simulink model "simulink_qbat_model"  (R2020b)
settings: Solver=ode4  StartTime=0.0  StopTime=1800  FixedStep=0.01  MaxStep=10  MinStep=0.1  RelTol=1e-3
model workspace (MAT data in the model file):
  air_initial_temperature = 25
  coolant_initial_temperature = 25
  electro_model = struct()
  fem_model = struct()
  heat_dt = 1
  initial_SOC = 0.8
  max_res = 0.001
  n_fv_gradient_subiters = 20
  n_subiters = 1
  number_of_electro_sub_steps = 10
  solids_initial_temperature = 25
libraries: muRata_US18650VTC4_201c01110_lib x5
settings Model: Creator=mkurzynka  LastModifiedBy=ŁukaszBazydło
settings SolverCC: InitialStep=0.1  SolverJacobianMethodControl=SparsePerturbation
settings DebuggingCC: ArithmeticOperatorsInVariantConditions=warning
settings ModelReferenceCC: UpdateModelReferenceTargets=Force
settings SFSimCC: CustomCodeUndefinedFunction=UseInterfaceOnly

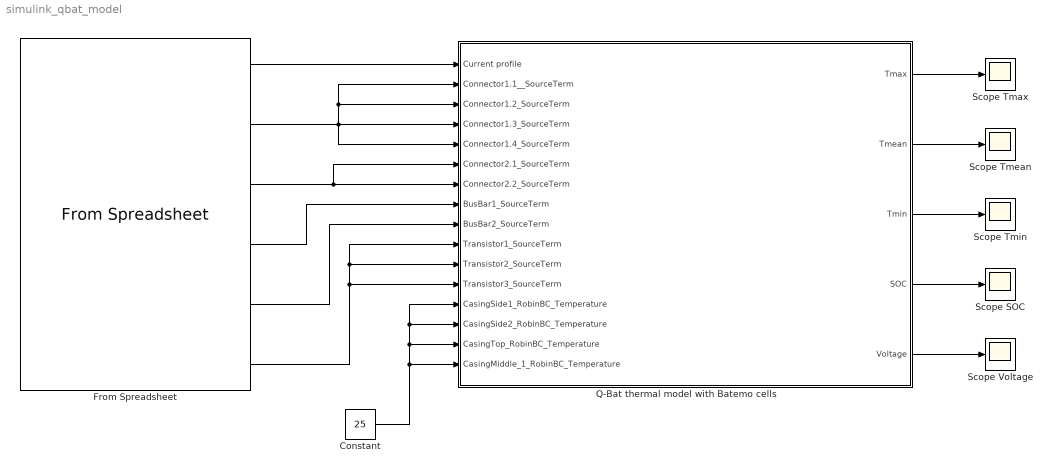
== system simulink_qbat_model ==
  Constant : Constant  Value=25
  From Spreadsheet : FromSpreadsheet  FileName=Simulink_losses2.xlsx  SheetName=Losses  Range=A1:G6362  OutDataTypeStr=double  SampleTime=0.1
  Q-Bat thermal model with Batemo cells : Subsystem  mask{dt=heat_dt, n_electro_substeps=number_of_electro_sub_steps, T_init_fem=solids_initial_temperature, T_init_th=coolant_initial_temperature, T_init_fv=air_initial_temperature, SOC_init=initial_SOC, n_subiters=n_subiters, n_maxres=max_res, FV_gradient_subiters=n_fv_gradient_subiters, solver_type=Iterative: PCG}
      mask prompts: dt "Temperature time step"; n_electro_substeps "Number of electro substeps"; T_init_fem "Initial temperature in solids"; T_init_th "Initial temperature in pipes"; T_init_fv "Initial temperature in air"; SOC_init "Initial SOC"; n_subiters "Number of thermal nonlinear subiterations"; n_maxres "Maxium error of thermal nonlinearity"; FV_gradient_subiters "Number of FV gradient subiterations"; solver_type "Solver type"
      mask TypeOptions solver_type: Direct | Iterative: PCG
  Scope SOC : Scope
  Scope Tmax : Scope
  Scope Tmean : Scope
  Scope Tmin : Scope
  Scope Voltage : Scope
  wires:
  Constant/1 -> Q-Bat thermal model with Batemo cells/13(CasingSide1_RobinBC_Temperature), Q-Bat thermal model with Batemo cells/14(CasingSide2_RobinBC_Temperature), Q-Bat thermal model with Batemo cells/15(CasingTop_RobinBC_Temperature), Q-Bat thermal model with Batemo cells/16(CasingMiddle_1_RobinBC_Temperature)
  Q-Bat thermal model with Batemo cells/1(Tmax) -> Scope Tmax/1
  Q-Bat thermal model with Batemo cells/2(Tmean) -> Scope Tmean/1
  Q-Bat thermal model with Batemo cells/3(Tmin) -> Scope Tmin/1
  Q-Bat thermal model with Batemo cells/5(Voltage) -> Scope Voltage/1
  Q-Bat thermal model with Batemo cells/4(SOC) -> Scope SOC/1
  From Spreadsheet/2 -> Q-Bat thermal model with Batemo cells/5(Connector1.4_SourceTerm), Q-Bat thermal model with Batemo cells/4(Connector1.3_SourceTerm), Q-Bat thermal model with Batemo cells/3(Connector1.2_SourceTerm), Q-Bat thermal model with Batemo cells/2(Connector1.1__SourceTerm)
  From Spreadsheet/3 -> Q-Bat thermal model with Batemo cells/7(Connector2.2_SourceTerm), Q-Bat thermal model with Batemo cells/6(Connector2.1_SourceTerm)
  From Spreadsheet/4 -> Q-Bat thermal model with Batemo cells/8(BusBar1_SourceTerm)
  From Spreadsheet/5 -> Q-Bat thermal model with Batemo cells/9(BusBar2_SourceTerm)
  From Spreadsheet/6 -> Q-Bat thermal model with Batemo cells/12(Transistor3_SourceTerm), Q-Bat thermal model with Batemo cells/11(Transistor2_SourceTerm), Q-Bat thermal model with Batemo cells/10(Transistor1_SourceTerm)
  From Spreadsheet/1 -> Q-Bat thermal model with Batemo cells/1(Current profile)

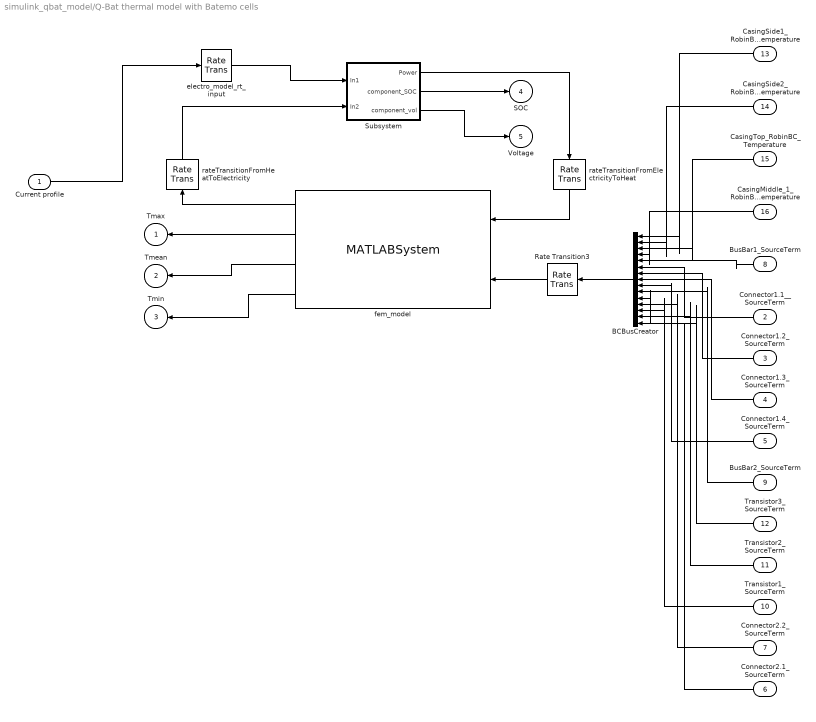
== system simulink_qbat_model/Q-Bat thermal model with Batemo cells ==
  Current profile : Inport
  Connector1.1__SourceTerm : Inport  Port=2
  Connector1.2_SourceTerm : Inport  Port=3
  Connector1.3_SourceTerm : Inport  Port=4
  Connector1.4_SourceTerm : Inport  Port=5
  Connector2.1_SourceTerm : Inport  Port=6
  Connector2.2_SourceTerm : Inport  Port=7
  BusBar1_SourceTerm : Inport  Port=8
  BusBar2_SourceTerm : Inport  Port=9
  Transistor1_SourceTerm : Inport  Port=10
  Transistor2_SourceTerm : Inport  Port=11
  Transistor3_SourceTerm : Inport  Port=12
  CasingSide1_RobinBC_Temperature : Inport  Port=13
  CasingSide2_RobinBC_Temperature : Inport  Port=14
  CasingTop_RobinBC_Temperature : Inport  Port=15
  CasingMiddle_1_RobinBC_Temperature : Inport  Port=16
  BCBusCreator : BusCreator  Inputs=15
  Rate Transition3 : RateTransition  InitialCondition=2  OutPortSampleTime=dt
  Subsystem : Subsystem
  electro_model_rt_input : RateTransition  InitialCondition=1  OutPortSampleTime=0.1
  fem_model : MATLABSystem  System=simulink_fem_model  T_init_fem=T_init_fem  T_init_th=T_init_th  T_init_fv=T_init_fv  dt=dt  max_res=n_maxres  max_sub_iter=n_subiters  n_fv_gradient_subiters=n_fv_gradient_subiters  solver_type=solver_type  SimulateUsing=Interpreted execution
      mask Type: simulink_fem_model
      mask Display:
      | disp('simulink_fem_model');
      | port_label('input',1,'ele_source_term');
      | port_label('input',2,'bus_input');
      | port_label('output',1,'fem_mean_temp');
      | port_label('output',2,'fem_max_temp_output');
      | port_label('output',3,'fem_mean_temp_output');
      | port_label('output',4,'fem_min_temp_output');
  rateTransitionFromElectricityToHeat : RateTransition  InitialCondition=0 * ones(5, 1)  OutPortSampleTime=dt
  rateTransitionFromHeatToElectricity : RateTransition  InitialCondition=T_init_fem * ones(5, 1)  OutPortSampleTime=0.1
  Tmax : Outport
  Tmean : Outport  Port=2
  Tmin : Outport  Port=3
  SOC : Outport  Port=4
  Voltage : Outport  Port=5
  wires:
  fem_model/1 -> rateTransitionFromHeatToElectricity/1
  electro_model_rt_input/1 -> Subsystem/1(In1)
  rateTransitionFromHeatToElectricity/1 -> Subsystem/2(In2)
  rateTransitionFromElectricityToHeat/1 -> fem_model/1
  Subsystem/1(Power) -> rateTransitionFromElectricityToHeat/1
  Rate Transition3/1 -> fem_model/2
  BCBusCreator/1 -> Rate Transition3/1
  Current profile/1 -> electro_model_rt_input/1
  fem_model/2 -> Tmax/1
  fem_model/3 -> Tmean/1
  fem_model/4 -> Tmin/1
  Subsystem/2(component_SOC) -> SOC/1
  Subsystem/3(component_vol) -> Voltage/1
  CasingSide1_RobinBC_Temperature/1 -> BCBusCreator/1
  CasingSide2_RobinBC_Temperature/1 -> BCBusCreator/2
  CasingTop_RobinBC_Temperature/1 -> BCBusCreator/3
  CasingMiddle_1_RobinBC_Temperature/1 -> BCBusCreator/4
  BusBar1_SourceTerm/1 -> BCBusCreator/5
  Connector1.1__SourceTerm/1 -> BCBusCreator/6
  Connector1.2_SourceTerm/1 -> BCBusCreator/7
  Connector1.3_SourceTerm/1 -> BCBusCreator/8
  Connector1.4_SourceTerm/1 -> BCBusCreator/9
  BusBar2_SourceTerm/1 -> BCBusCreator/10
  Connector2.1_SourceTerm/1 -> BCBusCreator/11
  Connector2.2_SourceTerm/1 -> BCBusCreator/12
  Transistor1_SourceTerm/1 -> BCBusCreator/13
  Transistor2_SourceTerm/1 -> BCBusCreator/14
  Transistor3_SourceTerm/1 -> BCBusCreator/15

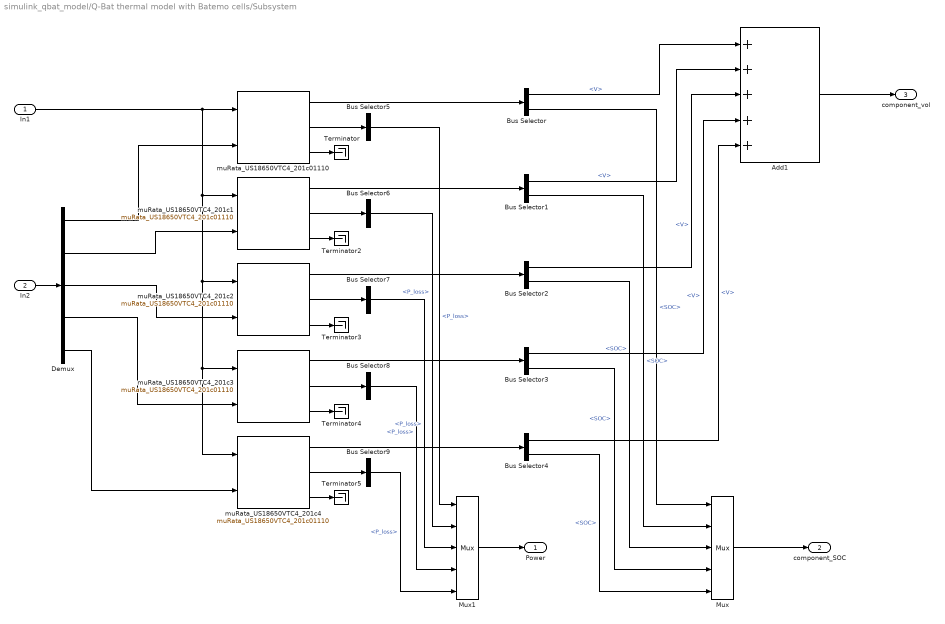
== system simulink_qbat_model/Q-Bat thermal model with Batemo cells/Subsystem ==
  In1 : Inport
  In2 : Inport  Port=2
  Add1 : Sum  Inputs=+++++
  Bus Selector{,1..4} (5 alike) : BusSelector  OutputSignals=V,SOC
  Bus Selector{5..9} (5 alike) : BusSelector  OutputSignals=P_loss
  Demux : Demux  Outputs=5
  Mux : Mux  Inputs=5
  Mux1 : Mux  Inputs=5
  Terminator{,2..5} (5 alike) : Terminator
  muRata_US18650VTC4_201c01110 : muRata_US18650VTC4_201c01110_lib/muRata_US18650VTC4_201c01110  Tag=muRata_US18650VTC4_201c01110  Description=Batemo Battery Model of a single cell of type BatteryName.  select_initial_SOC_OCV=SOC  SOC_0=100.0  V_ocv_0=3.5  T_inner_0=25  N_serial=1  N_parallel=1  select_input_I_V=Current Input  select_input_J_T=Temperature Input  enable_addon_ap=off  select_aging_scenario=none  k_C_fu=100  k_loss_fu=100  dummy=100  k_C_an=0  k_C_ca=0  k_C_li=0  k_C_an1=0  k_C_ca1=0  k_C_x=0  k_loss_an=0  k_loss_ca=0  k_loss_x=0  k_loss_an1=0  k_loss_ca1=0  k_loss_x1=0  enable_addon_pe=on  enable_addon_ac=off  enable_addon_lbc=off  enable_addon_lpe=off  enable_addon_lac=off  tau_filter=1e-07  T_inner_feedthrough=off
  muRata_US18650VTC4_201c{1..4} (4 alike) : muRata_US18650VTC4_201c01110_lib/muRata_US18650VTC4_201c01110  Tag=muRata_US18650VTC4_201c01110  Description=Batemo Battery Model of a single cell of type BatteryName.  select_initial_SOC_OCV=SOC  SOC_0=100.0  V_ocv_0=3.5  T_inner_0=25  N_serial=1  N_parallel=1  select_input_I_V=Current Input  select_input_J_T=Temperature Input  enable_addon_ap=off  select_aging_scenario=none  k_C_fu=100  k_loss_fu=100  dummy=100  k_C_an=0  k_C_ca=0  k_C_li=0  k_C_an1=0  k_C_ca1=0  k_C_x=0  k_loss_an=0  k_loss_ca=0  k_loss_x=0  k_loss_an1=0  k_loss_ca1=0  k_loss_x1=0  enable_addon_pe=on  enable_addon_ac=off  enable_addon_lbc=off  enable_addon_lpe=off  enable_addon_lac=off  tau_filter=1e-07  T_inner_feedthrough=off
  Power : Outport
  component_SOC : Outport  Port=2
  component_vol : Outport  Port=3
  wires:
  In1/1 -> muRata_US18650VTC4_201c01110/1, muRata_US18650VTC4_201c1/1, muRata_US18650VTC4_201c2/1, muRata_US18650VTC4_201c3/1, muRata_US18650VTC4_201c4/1
  muRata_US18650VTC4_201c01110/3 -> Terminator/1
  muRata_US18650VTC4_201c1/3 -> Terminator2/1
  muRata_US18650VTC4_201c2/3 -> Terminator3/1
  muRata_US18650VTC4_201c3/3 -> Terminator4/1
  muRata_US18650VTC4_201c4/3 -> Terminator5/1
  Add1/1 -> component_vol/1
  Mux/1 -> component_SOC/1
  In2/1 -> Demux/1
  Demux/1 -> muRata_US18650VTC4_201c01110/2
  Demux/2 -> muRata_US18650VTC4_201c1/2
  Demux/3 -> muRata_US18650VTC4_201c2/2
  Demux/4 -> muRata_US18650VTC4_201c3/2
  Demux/5 -> muRata_US18650VTC4_201c4/2
  muRata_US18650VTC4_201c01110/1 -> Bus Selector/1
  muRata_US18650VTC4_201c1/1 -> Bus Selector1/1
  muRata_US18650VTC4_201c2/1 -> Bus Selector2/1
  muRata_US18650VTC4_201c3/1 -> Bus Selector3/1
  muRata_US18650VTC4_201c4/1 -> Bus Selector4/1
  muRata_US18650VTC4_201c01110/2 -> Bus Selector5/1
  muRata_US18650VTC4_201c1/2 -> Bus Selector6/1
  muRata_US18650VTC4_201c2/2 -> Bus Selector7/1
  muRata_US18650VTC4_201c3/2 -> Bus Selector8/1
  muRata_US18650VTC4_201c4/2 -> Bus Selector9/1
  Bus Selector9/1 -> Mux1/5  "<P_loss>"
  Bus Selector8/1 -> Mux1/4  "<P_loss>"
  Bus Selector7/1 -> Mux1/3  "<P_loss>"
  Bus Selector6/1 -> Mux1/2  "<P_loss>"
  Bus Selector5/1 -> Mux1/1  "<P_loss>"
  Bus Selector/1 -> Add1/1  "<V>"
  Bus Selector1/1 -> Add1/2  "<V>"
  Bus Selector2/1 -> Add1/3  "<V>"
  Bus Selector3/1 -> Add1/4  "<V>"
  Bus Selector4/1 -> Add1/5  "<V>"
  Bus Selector4/2 -> Mux/5  "<SOC>"
  Bus Selector3/2 -> Mux/4  "<SOC>"
  Bus Selector2/2 -> Mux/3  "<SOC>"
  Bus Selector1/2 -> Mux/2  "<SOC>"
  Bus Selector/2 -> Mux/1  "<SOC>"
  Mux1/1 -> Power/1
